simulink model "Flexible_Fishtail_CTLSys"  (R2022b)
settings: Solver=FixedStepAuto  StartTime=0.0  StopTime=12  FixedStep=5e-5  RelTol=1e-3
libraries: slpidlib x3, spsMeanLib x1, rllib x1
settings Model: Creator=acer  LastModifiedBy=10640
settings SolverCC: AlgebraicLoopSolver=TrustRegion
settings DataIOCC: ReturnWorkspaceOutputs=off
settings OptimizationCC: DefaultParameterBehavior=Inlined  UseDivisionForNetSlopeComputation=on  GainParamInheritBuiltInType=on  UseFloatMulNetSlope=on  InlineInvariantSignals=on  EnhancedBackFolding=on  PassReuseOutputArgsAs=Individual arguments  ZeroExternalMemoryAtStartup=off  ZeroInternalMemoryAtStartup=off  EfficientFloat2IntCast=on  OptimizeBlockOrder=speed  DifferentSizesBufferReuse=on  OptimizationCustomize=off  EfficientTunableParamExpr=on
settings DebuggingCC: ParameterTunabilityLossMsg=error  UnconnectedInputMsg=warning  UnconnectedOutputMsg=warning  UnconnectedLineMsg=warning  PregeneratedLibrarySubsystemCodeDiagnostic=none  SFMachineParentedDataDiag=warning  ArithmeticOperatorsInVariantConditions=warning
settings HardwareCC: ProdLongLongMode=on
settings ModelReferenceCC: EnableRefExpFcnMdlSchedulingChecks=on
settings SFSimCC: SimUseLocalCustomCode=off  MATLABDynamicMemAlloc=off  CustomCodeUndefinedFunction=UseInterfaceOnly
settings RTWCC: Description=Embedded Coder  SystemTargetFile=ert.tlc  TemplateMakefile=ert_default_tmf  GenerateReport=on  RTWUseLocalCustomCode=off  LaunchReport=on
settings CodeAppCC: ForceParamTrailComments=on  IgnoreCustomStorageClasses=off  OperatorAnnotations=on  SimulinkDataObjDesc=on  SFDataObjDesc=on  InsertBlockDesc=on
settings ERTTargetCC: TargetLangStandard=C99 (ISO)  GenerateSampleERTMain=on  InlinedParameterPlacement=NonHierarchical  ERTCustomFileTemplate=example_file_process.tlc

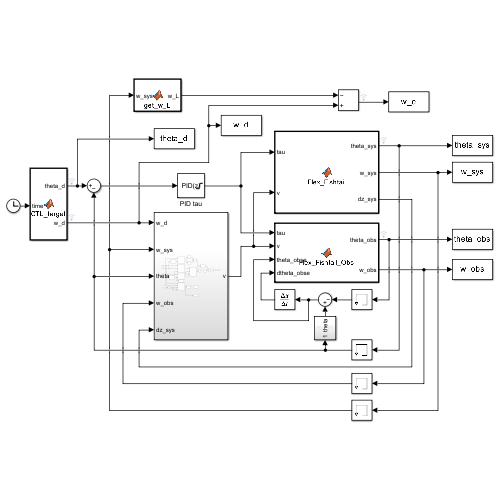
[thumbnail: Simulink's stored preview of the top-level diagram]
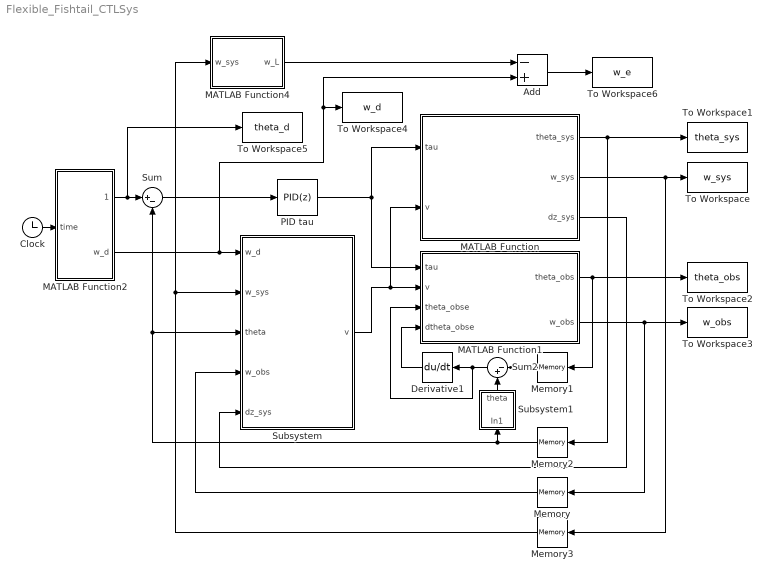
== system Flexible_Fishtail_CTLSys ==
  Add : Sum  Inputs=-+
  Clock : Clock
  Derivative1 : Derivative
  MATLAB Function : MATLAB Function  TreatAsAtomicUnit=on
  MATLAB Function1 : MATLAB Function  TreatAsAtomicUnit=on
  MATLAB Function2 : MATLAB Function  TreatAsAtomicUnit=on
  MATLAB Function4 : MATLAB Function  TreatAsAtomicUnit=on
  Memory{,1..3} (4 alike) : Memory
  PID tau : slpidlib/PID Controller  Controller=PID  Form=Parallel  TimeDomain=Discrete-time  UseExternalTs=off  SampleTime=-1  IntegratorMethod=Forward Euler  FilterMethod=Forward Euler  ControllerParametersSource=internal  P=1.5  I=50  UseKiTs=off  D=0.01  N=100  UseFilter=off  TunerSelectOption=Transfer Function Based (PID Tuner App)  InitialConditionSource=internal  InitialConditionForIntegrator=0  InitialConditionForFilter=0  DifferentiatorICPrevScaledInput=0  ExternalReset=none  TrackingMode=off  Kt=1  LimitOutput=on  SatLimitsSource=internal  UpperSaturationLimit=0.5  LowerSaturationLimit=-0.5  LinearizeAsGain=on  AntiWindupMode=none  Kb=1  LimitIntegrator=off  UpperIntegratorSaturationLimit=inf  LowerIntegratorSaturationLimit=-inf  POutMin=[]  POutMax=[]  IOutMin=[]  IOutMax=[]  DOutMin=[]  DOutMax=[]  NOutMin=[]  NOutMax=[]  SumOutMin=[]  SumOutMax=[]  SaturationOutMin=[]  SaturationOutMax=[]  PParamMin=[]  PParamMax=[]  IParamMin=[]  IParamMax=[]  DParamMin=[]  DParamMax=[]  NParamMin=[]  NParamMax=[]  KbParamMin=[]  KbParamMax=[]  KtParamMin=[]  KtParamMax=[]  KbOutMin=[]  KbOutMax=[]  KtOutMin=[]  KtOutMax=[]  IntegratorOutMin=[]  IntegratorOutMax=[]  FilterOutMin=[]  FilterOutMax=[]  SumI1OutMin=[]  SumI1OutMax=[]  SumI2OutMin=[]  SumI2OutMax=[]  SumI3OutMin=[]  SumI3OutMax=[]  SumI4OutMin=[]  SumI4OutMax=[]  SumDOutMin=[]  SumDOutMax=[]  DifferentiatorOutMin=[]  DifferentiatorOutMax=[]  FilterDiffOutCoefMin=[]  FilterDiffOutCoefMax=[]  ReciprocalOutMin=[]  ReciprocalOutMax=[]  SumDenOutMin=[]  SumDenOutMax=[]  SumNumOutMin=[]  SumNumOutMax=[]  DivideOutMin=[]  DivideOutMax=[]  UdiffTsProdOutMin=[]  UdiffTsProdOutMax=[]  NTsProdOutMin=[]  NTsProdOutMax=[]  UintegralTsProdOutMin=[]  UintegralTsProdOutMax=[]  UngainTsProdOutMin=[]  UngainTsProdOutMax=[]  ClampingZeroOutDataTypeStr=Inherit: Inherit via back propagation  ClampingZeroOutMin=[]  ClampingZeroOutMax=[]  FilterDenConstantOutDataTypeStr=Inherit: Inherit via back propagation  FilterDenConstantOutMin=[]  FilterDenConstantOutMax=[]  PCopyOutDataTypeStr=Inherit: Inherit via back propagation  PCopyOutMin=[]  PCopyOutMax=[]  NCopyOutDataTypeStr=Inherit: Inherit via back propagation  NCopyOutMin=[]  NCopyOutMax=[]  IntegratorContinuousStateAttributes=''  IntegratorStateMustResolveToSignalObject=off  IntegratorRTWStateStorageClass=Auto  FilterContinuousStateAttributes=''  FilterStateMustResolveToSignalObject=off  FilterRTWStateStorageClass=Auto  ParallelPVariant=InternalParameters  IdealPVariant=Disabled  IVariant=InternalParameters  DVariant=InternalParameters  IntegratorVariant=Discrete  SatVariant=Enabled  AWVariant=Passthrough  PCopyVariant=Disabled  TRVariant=Disabled  FdbkBlocksVariant=Forward  IdealPFdbkVariant=Disabled  SatFdbkVariant=Disabled  DerivativeFilterVariant=Differentiator  NVariant=Passthrough  NCopyVariant=Disabled_SignalSpec  FilterICVariant=InternalICsDifferentiator  IntegratorICVariant=InternalICs  ExternalResetVariant=Disabled  TRSumVariant=Passthrough  SumFdbkVariant=Disabled  SumVariant=Sum_PID  TsampFilterVariant=InternalTs  TsampNgainVariant=Passthrough  TsampIntegralVariant=Passthrough  ExternalSaturationOutDataTypeStr=Inherit: Same as second input
  Subsystem : Subsystem
  Subsystem1 : Subsystem
  Sum : Sum  Inputs=|+-
  Sum2 : Sum  Inputs=|-+
  To Workspace : ToWorkspace  VariableName=w_sys  SampleTime=-1
  To Workspace1 : ToWorkspace  VariableName=theta_sys  SampleTime=-1
  To Workspace2 : ToWorkspace  VariableName=theta_obs  SampleTime=-1
  To Workspace3 : ToWorkspace  VariableName=w_obs  SampleTime=-1
  To Workspace4 : ToWorkspace  VariableName=w_d  SampleTime=-1
  To Workspace5 : ToWorkspace  VariableName=theta_d  SampleTime=-1
  To Workspace6 : ToWorkspace  VariableName=w_e  SampleTime=-1
  wires:
  Clock/1 -> MATLAB Function2/1(time)
  MATLAB Function2/1(theta_d) -> To Workspace5/1, Sum/1
  Sum/1 -> PID tau/1
  Derivative1/1 -> MATLAB Function1/4(dtheta_obse)
  MATLAB Function/1(theta_sys) -> Memory2/1, To Workspace1/1
  Sum2/1 -> Derivative1/1, MATLAB Function1/3(theta_obse)
  MATLAB Function2/2(w_d) -> Add/2, To Workspace4/1, Subsystem/1(w_d)
  MATLAB Function1/2(w_obs) -> To Workspace3/1, Memory/1
  MATLAB Function1/1(theta_obs) -> To Workspace2/1, Memory1/1
  Memory1/1 -> Sum2/1
  PID tau/1 -> MATLAB Function/1(tau), MATLAB Function1/1(tau)
  Subsystem/1(v) -> MATLAB Function/2(v), MATLAB Function1/2(v)
  MATLAB Function/2(w_sys) -> Memory3/1, To Workspace/1
  Memory/1 -> Subsystem/4(w_obs)
  Memory2/1 -> Sum/2, Subsystem/3(theta), Subsystem1/1(In1)
  Subsystem1/1(theta) -> Sum2/2
  Memory3/1 -> MATLAB Function4/1(w_sys), Subsystem/2(w_sys)
  MATLAB Function4/1(w_L) -> Add/1
  Add/1 -> To Workspace6/1
  MATLAB Function/3(dz_sys) -> Subsystem/5(dz_sys)

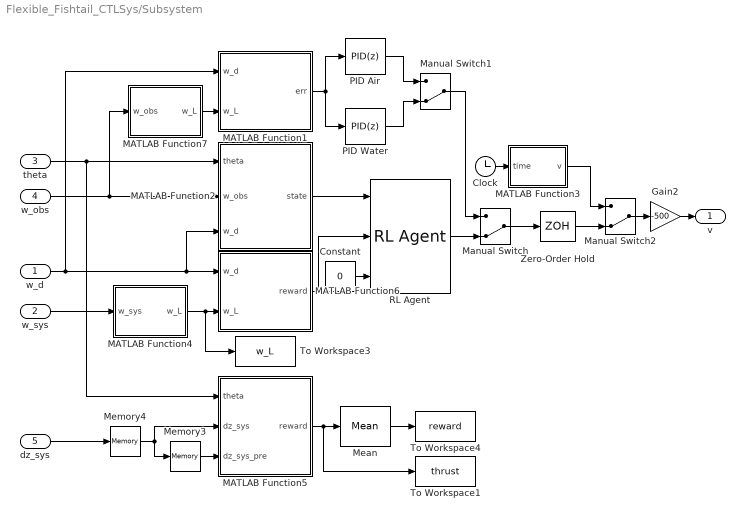
== system Flexible_Fishtail_CTLSys/Subsystem ==
  w_d : Inport
  w_sys : Inport  Port=2
  theta : Inport  Port=3
  w_obs : Inport  Port=4
  dz_sys : Inport  Port=5
  Clock : Clock
  Constant : Constant  Value=0
  Gain2 : Gain  Gain=-500
  MATLAB Function1 : MATLAB Function  TreatAsAtomicUnit=on
  MATLAB Function2 : MATLAB Function  TreatAsAtomicUnit=on
  MATLAB Function3 : MATLAB Function  TreatAsAtomicUnit=on
  MATLAB Function4 : MATLAB Function  TreatAsAtomicUnit=on
  MATLAB Function5 : MATLAB Function  TreatAsAtomicUnit=on
  MATLAB Function6 : MATLAB Function  TreatAsAtomicUnit=on
  MATLAB Function7 : MATLAB Function  TreatAsAtomicUnit=on
  Manual Switch : ManualSwitch  CurrentSetting=0
  Manual Switch1 : ManualSwitch  CurrentSetting=0
  Manual Switch2 : ManualSwitch  CurrentSetting=0
  Mean : spsMeanLib/Mean  Freq=0.5  Vinit=0  Ts=5e-5
  Memory3 : Memory
  Memory4 : Memory
  PID Air : slpidlib/PID Controller  Controller=PID  Form=Parallel  TimeDomain=Discrete-time  UseExternalTs=off  SampleTime=-1  IntegratorMethod=Forward Euler  FilterMethod=Forward Euler  ControllerParametersSource=internal  P=0.00005  I=0.02  UseKiTs=off  D=0  N=100  UseFilter=off  TunerSelectOption=Transfer Function Based (PID Tuner App)  InitialConditionSource=internal  InitialConditionForIntegrator=0  InitialConditionForFilter=0  DifferentiatorICPrevScaledInput=0  ExternalReset=none  TrackingMode=off  Kt=1  LimitOutput=on  SatLimitsSource=internal  UpperSaturationLimit=1  LowerSaturationLimit=-1  LinearizeAsGain=on  AntiWindupMode=none  Kb=1  LimitIntegrator=off  UpperIntegratorSaturationLimit=inf  LowerIntegratorSaturationLimit=-inf  POutMin=[]  POutMax=[]  IOutMin=[]  IOutMax=[]  DOutMin=[]  DOutMax=[]  NOutMin=[]  NOutMax=[]  SumOutMin=[]  SumOutMax=[]  SaturationOutMin=[]  SaturationOutMax=[]  PParamMin=[]  PParamMax=[]  IParamMin=[]  IParamMax=[]  DParamMin=[]  DParamMax=[]  NParamMin=[]  NParamMax=[]  KbParamMin=[]  KbParamMax=[]  KtParamMin=[]  KtParamMax=[]  KbOutMin=[]  KbOutMax=[]  KtOutMin=[]  KtOutMax=[]  IntegratorOutMin=[]  IntegratorOutMax=[]  FilterOutMin=[]  FilterOutMax=[]  SumI1OutMin=[]  SumI1OutMax=[]  SumI2OutMin=[]  SumI2OutMax=[]  SumI3OutMin=[]  SumI3OutMax=[]  SumI4OutMin=[]  SumI4OutMax=[]  SumDOutMin=[]  SumDOutMax=[]  DifferentiatorOutMin=[]  DifferentiatorOutMax=[]  FilterDiffOutCoefMin=[]  FilterDiffOutCoefMax=[]  ReciprocalOutMin=[]  ReciprocalOutMax=[]  SumDenOutMin=[]  SumDenOutMax=[]  SumNumOutMin=[]  SumNumOutMax=[]  DivideOutMin=[]  DivideOutMax=[]  UdiffTsProdOutMin=[]  UdiffTsProdOutMax=[]  NTsProdOutMin=[]  NTsProdOutMax=[]  UintegralTsProdOutMin=[]  UintegralTsProdOutMax=[]  UngainTsProdOutMin=[]  UngainTsProdOutMax=[]  ClampingZeroOutDataTypeStr=Inherit: Inherit via back propagation  ClampingZeroOutMin=[]  ClampingZeroOutMax=[]  FilterDenConstantOutDataTypeStr=Inherit: Inherit via back propagation  FilterDenConstantOutMin=[]  FilterDenConstantOutMax=[]  PCopyOutDataTypeStr=Inherit: Inherit via back propagation  PCopyOutMin=[]  PCopyOutMax=[]  NCopyOutDataTypeStr=Inherit: Inherit via back propagation  NCopyOutMin=[]  NCopyOutMax=[]  IntegratorContinuousStateAttributes=''  IntegratorStateMustResolveToSignalObject=off  IntegratorRTWStateStorageClass=Auto  FilterContinuousStateAttributes=''  FilterStateMustResolveToSignalObject=off  FilterRTWStateStorageClass=Auto  ParallelPVariant=InternalParameters  IdealPVariant=Disabled  IVariant=InternalParameters  DVariant=InternalParameters  IntegratorVariant=Discrete  SatVariant=Enabled  AWVariant=Passthrough  PCopyVariant=Disabled  TRVariant=Disabled  FdbkBlocksVariant=Forward  IdealPFdbkVariant=Disabled  SatFdbkVariant=Disabled  DerivativeFilterVariant=Differentiator  NVariant=Passthrough  NCopyVariant=Disabled_SignalSpec  FilterICVariant=InternalICsDifferentiator  IntegratorICVariant=InternalICs  ExternalResetVariant=Disabled  TRSumVariant=Passthrough  SumFdbkVariant=Disabled  SumVariant=Sum_PID  TsampFilterVariant=InternalTs  TsampNgainVariant=Passthrough  TsampIntegralVariant=Passthrough  ExternalSaturationOutDataTypeStr=Inherit: Same as second input
  PID Water : slpidlib/PID Controller  Controller=PID  Form=Parallel  TimeDomain=Discrete-time  UseExternalTs=off  SampleTime=-1  IntegratorMethod=Forward Euler  FilterMethod=Forward Euler  ControllerParametersSource=internal  P=0.0001  I=0.035  UseKiTs=off  D=0.00000001  N=100  UseFilter=off  TunerSelectOption=Transfer Function Based (PID Tuner App)  InitialConditionSource=internal  InitialConditionForIntegrator=0  InitialConditionForFilter=0  DifferentiatorICPrevScaledInput=0  ExternalReset=none  TrackingMode=off  Kt=1  LimitOutput=on  SatLimitsSource=internal  UpperSaturationLimit=1  LowerSaturationLimit=-1  LinearizeAsGain=on  AntiWindupMode=none  Kb=1  LimitIntegrator=off  UpperIntegratorSaturationLimit=inf  LowerIntegratorSaturationLimit=-inf  POutMin=[]  POutMax=[]  IOutMin=[]  IOutMax=[]  DOutMin=[]  DOutMax=[]  NOutMin=[]  NOutMax=[]  SumOutMin=[]  SumOutMax=[]  SaturationOutMin=[]  SaturationOutMax=[]  PParamMin=[]  PParamMax=[]  IParamMin=[]  IParamMax=[]  DParamMin=[]  DParamMax=[]  NParamMin=[]  NParamMax=[]  KbParamMin=[]  KbParamMax=[]  KtParamMin=[]  KtParamMax=[]  KbOutMin=[]  KbOutMax=[]  KtOutMin=[]  KtOutMax=[]  IntegratorOutMin=[]  IntegratorOutMax=[]  FilterOutMin=[]  FilterOutMax=[]  SumI1OutMin=[]  SumI1OutMax=[]  SumI2OutMin=[]  SumI2OutMax=[]  SumI3OutMin=[]  SumI3OutMax=[]  SumI4OutMin=[]  SumI4OutMax=[]  SumDOutMin=[]  SumDOutMax=[]  DifferentiatorOutMin=[]  DifferentiatorOutMax=[]  FilterDiffOutCoefMin=[]  FilterDiffOutCoefMax=[]  ReciprocalOutMin=[]  ReciprocalOutMax=[]  SumDenOutMin=[]  SumDenOutMax=[]  SumNumOutMin=[]  SumNumOutMax=[]  DivideOutMin=[]  DivideOutMax=[]  UdiffTsProdOutMin=[]  UdiffTsProdOutMax=[]  NTsProdOutMin=[]  NTsProdOutMax=[]  UintegralTsProdOutMin=[]  UintegralTsProdOutMax=[]  UngainTsProdOutMin=[]  UngainTsProdOutMax=[]  ClampingZeroOutDataTypeStr=Inherit: Inherit via back propagation  ClampingZeroOutMin=[]  ClampingZeroOutMax=[]  FilterDenConstantOutDataTypeStr=Inherit: Inherit via back propagation  FilterDenConstantOutMin=[]  FilterDenConstantOutMax=[]  PCopyOutDataTypeStr=Inherit: Inherit via back propagation  PCopyOutMin=[]  PCopyOutMax=[]  NCopyOutDataTypeStr=Inherit: Inherit via back propagation  NCopyOutMin=[]  NCopyOutMax=[]  IntegratorContinuousStateAttributes=''  IntegratorStateMustResolveToSignalObject=off  IntegratorRTWStateStorageClass=Auto  FilterContinuousStateAttributes=''  FilterStateMustResolveToSignalObject=off  FilterRTWStateStorageClass=Auto  ParallelPVariant=InternalParameters  IdealPVariant=Disabled  IVariant=InternalParameters  DVariant=InternalParameters  IntegratorVariant=Discrete  SatVariant=Enabled  AWVariant=Passthrough  PCopyVariant=Disabled  TRVariant=Disabled  FdbkBlocksVariant=Forward  IdealPFdbkVariant=Disabled  SatFdbkVariant=Disabled  DerivativeFilterVariant=Differentiator  NVariant=Passthrough  NCopyVariant=Disabled_SignalSpec  FilterICVariant=InternalICsDifferentiator  IntegratorICVariant=InternalICs  ExternalResetVariant=Disabled  TRSumVariant=Passthrough  SumFdbkVariant=Disabled  SumVariant=Sum_PID  TsampFilterVariant=InternalTs  TsampNgainVariant=Passthrough  TsampIntegralVariant=Passthrough  ExternalSaturationOutDataTypeStr=Inherit: Same as second input
  RL Agent : rllib/RL Agent  Agent=agent  ExternalActionAsInput=off  ProvideLastAction=off  ProvideCumRwd=off  TreatAsDirectFeedthrough=on  UseStrictObservationDataTypes=off
  To Workspace1 : ToWorkspace  VariableName=thrust  SampleTime=-1
  To Workspace3 : ToWorkspace  VariableName=w_L  SampleTime=-1
  To Workspace4 : ToWorkspace  VariableName=reward  SampleTime=-1
  Zero-Order Hold : ZeroOrderHold  SampleTime=20e-3
  v : Outport  VectorParamsAs1DForOutWhenUnconnected=off
  wires:
  Memory3/1 -> MATLAB Function5/3(dz_sys_pre)
  Memory4/1 -> Memory3/1, MATLAB Function5/2(dz_sys)
  Constant/1 -> RL Agent/3
  w_d/1 -> MATLAB Function1/1(w_d), MATLAB Function2/3(w_d), MATLAB Function6/1(w_d)
  w_sys/1 -> MATLAB Function4/1(w_sys)
  w_obs/1 -> MATLAB Function7/1(w_obs), MATLAB Function2/2(w_obs)
  RL Agent/1 -> Manual Switch/2
  MATLAB Function1/1(err) -> PID Water/1, PID Air/1
  MATLAB Function2/1(state) -> RL Agent/1
  MATLAB Function6/1(reward) -> RL Agent/2
  Gain2/1 -> v/1
  Mean/1 -> To Workspace4/1
  PID Air/1 -> Manual Switch1/1
  Manual Switch1/1 -> Manual Switch/1
  PID Water/1 -> Manual Switch1/2
  Clock/1 -> MATLAB Function3/1(time)
  MATLAB Function4/1(w_L) -> To Workspace3/1, MATLAB Function6/2(w_L)
  MATLAB Function7/1(w_L) -> MATLAB Function1/2(w_L)
  Manual Switch/1 -> Zero-Order Hold/1
  Zero-Order Hold/1 -> Manual Switch2/2
  MATLAB Function3/1(v) -> Manual Switch2/1
  Manual Switch2/1 -> Gain2/1
  MATLAB Function5/1(reward) -> To Workspace1/1, Mean/1
  dz_sys/1 -> Memory4/1
  theta/1 -> MATLAB Function5/1(theta), MATLAB Function2/1(theta)

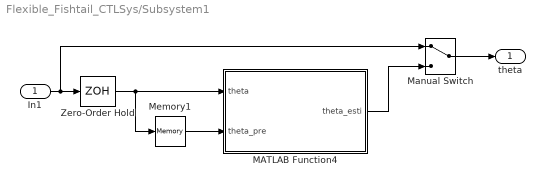
== system Flexible_Fishtail_CTLSys/Subsystem1 ==
  In1 : Inport
  MATLAB Function4 : MATLAB Function  TreatAsAtomicUnit=on
  Manual Switch : ManualSwitch
  Memory1 : Memory
  Zero-Order Hold : ZeroOrderHold  SampleTime=30e-3
  theta : Outport
  wires:
  In1/1 -> Manual Switch/1, Zero-Order Hold/1
  Zero-Order Hold/1 -> MATLAB Function4/1(theta), Memory1/1
  Memory1/1 -> MATLAB Function4/2(theta_pre)
  MATLAB Function4/1(theta_esti) -> Manual Switch/2
  Manual Switch/1 -> theta/1

== matlab function Flexible_Fishtail_CTLSys/Subsystem/MATLAB Function7 ==
  data: w_obs input; w_L output
function w_L = get_w_L(w_obs)
    w_L = w_obs(end);
end

== matlab function Flexible_Fishtail_CTLSys/Subsystem/MATLAB Function4 ==
  data: w_sys input; w_L output
function w_L = get_w_L(w_sys)
    w_L = w_sys(end);
end

== matlab function Flexible_Fishtail_CTLSys/MATLAB Function4 ==
  data: w_sys input; w_L output
function w_L = get_w_L(w_sys)
    w_L = w_sys(end);
end

== matlab function Flexible_Fishtail_CTLSys/MATLAB Function1 ==
  settings: updateMethod=DISCRETE
  data: theta_obs output; w_obs output; tau input; v input; theta_obse input; dtheta_obse input
function [theta_obs, w_obs] = Flex_Fishtail_Obs(tau, v, theta_obse, dtheta_obse)
    %***********************************************************
    persistent angle_obs;
    persistent angle_obs_pre;
    persistent omega_obs;
    persistent omega_obs_pre;
    
    if isempty(angle_obs)
        angle_obs = 10/180*pi;
        angle_obs_pre = angle_obs;
        omega_obs = [ 0; 0; 0; 0; 0; 0; 0; 0; 0; 0; 0; 0; 0; 0; 0; 0; 0; 0; 0];
        omega_obs_pre = omega_obs;
    end
    
    dt = 5e-5;
    
    k_obs=0.015;
    gamma_obs=15;

    Ih=1e-6;
    c=0.1;
    rhow=1000;
    Caf=0.05;
    Cdf=1.2;

    L=0.17;
    nx=19;
    dx=L/(nx-1);
    bx1=round(0.03/dx)+1;
    bx2=round(0.14/dx)+1;
    xL0=round(0.0365/dx)+1;
    xL1=round(0.1375/dx)+1;

    d=0.0002;
    Eb=230e9;
    rhob=1760;
    dmfc=0.0003;
    bmfc=0.014;
    Emfc=30.336e9;
    rhoc=5440;
    d33=460e-12;
    deltad=0.5e-3;
    b=zeros(nx,1);
    EI=zeros(nx,1);
    rho_w=zeros(nx,1);
    cw=zeros(nx,1);
    rho=zeros(nx,1);
    R=zeros(nx,1);

    elecmech=1.66*2*Emfc*bmfc*d33*(d*dmfc+dmfc^2)/(2*deltad);

    for i=1:nx
        if i<bx1
            b(i)=0.04;
        elseif i>bx2
            b(i)=2.3*(i-bx2)*dx+0.026;
        else
            b(i)=2*sqrt(0.96375^2-((i-bx1)*dx)^2)-1.8875;
        end
    end

    for i=1:nx
        if i<xL0
            R(i)=0;
        elseif i>xL1
            R(i)=0;
        else
            R(i)=1;
        end
        EI(i)=R(i)*Emfc*bmfc*(2*dmfc^3/3+d*dmfc^2+0.5*dmfc*d^2)+Eb*d^3*b(i)/12;
        rho_w(i)=0.25*pi*rhow*b(i)^2*Caf;
        cw(i)=0.5*rhow*b(i)*Cdf;
        rho(i)=R(i)*dmfc*bmfc*2*rhoc+d*b(i)*rhob+rho_w(i);
    end
    
    theta=angle_obs;
    theta_pre=angle_obs_pre;
    w=omega_obs;
    w_pre=omega_obs_pre;

    w_new=zeros(nx,1);
    dw=zeros(nx,1);
    dz=zeros(nx,1);
    wxx=zeros(nx,1);
    EIwxx=zeros(nx,1);
    MR=zeros(nx,1);
        
    wxx0=(w(bx1+1)-2*w(bx1)+w(bx1-1))/dx^2;
    theta_new=2*theta-theta_pre+(EI(1)*wxx0+tau...
              +k_obs*(dtheta_obse+gamma_obs*theta_obse)...
              +gamma_obs*Ih*dtheta_obse)*dt^2/Ih;
    
    dtheta=(theta-theta_pre)/dt;
    ddtheta=(theta_new-2*theta+theta_pre)/dt^2;
    for i=1:nx
        dw(i)=(w(i)-w_pre(i))/dt;
        dz(i)=(i-1)*dx*dtheta+dw(i);
    end
    for i=2:nx-1
        wxx(i)=(w(i+1)-2*w(i)+w(i-1))/dx^2;
        EIwxx(i)=EI(i)*wxx(i);
        MR(i)=elecmech*v*R(i);
    end
    
    %Firstly, 1≤i≤bx1
    for i=1:bx1
        w_new(i)=0;
    end
    
    %Secondly, bx1≤i≤nx-2
    for i=bx1+1:nx-2
        EIwxxxx=(EIwxx(i+1)-2*EIwxx(i)+EIwxx(i-1))/dx^2;
        MRxx=(MR(i+1)-2*MR(i)+MR(i-1))/dx^2;
        w_new(i)=2*w(i)-w_pre(i)+(MRxx-EIwxxxx-c*dz(i)...
...%                  -cw(i)*abs(dz(i))*dz(i)...
                 -rho(i)*(i-1)*dx*ddtheta)*dt^2/rho(i);
    end
    %Thirdly, i=nx-1
    EIwxxxx1=EI(nx-1)*(-2*w(nx)+5*w(nx-1)-4*w(nx-2)+w(nx-3))/dx^4;
    w_new(nx-1)=2*w(nx-1)-w_pre(nx-1)+(-EIwxxxx1-c*dz(nx-1)...
...%                 -cw(nx-1)*abs(dz(nx-1))*dz(nx-1)...
                -rho(nx-1)*(nx-2)*dx*ddtheta)*dt^2/rho(nx-1);
    %Finally, i=nx
    EIwxxxx2=EI(nx)*(2*w(nx)-3*w(nx-1)+w(nx-2))/dx^4;
    w_new(nx)=2*w(nx)-w_pre(nx)+(-EIwxxxx2-c*dz(nx)...
...%                 -cw(nx)*abs(dz(nx))*dz(nx)...
                -rho(nx)*(nx-1)*dx*ddtheta)*dt^2/rho(nx);
       
    angle_obs=theta_new;
    angle_obs_pre=theta;
    omega_obs=w_new;
    omega_obs_pre=w;
    
    theta_obs=theta_new;
    w_obs=w_new;
    
end

== matlab function Flexible_Fishtail_CTLSys/MATLAB Function ==
  settings: updateMethod=DISCRETE
  data: theta_sys output; w_sys output; tau input; v input; dz_sys output
function [theta_sys, w_sys, dz_sys] = Flex_Fishtail(tau, v)
    %***********************************************************
    persistent angle;
    persistent angle_pre;
    persistent omega;
    persistent omega_pre;
    
    if isempty(angle)
%         angle = (2 * rand() - 1)*5/180*pi;
        angle = 10/180*pi;
        angle_pre = angle;
%         omega = [ 0; 0; -0.0002; -0.0004;
%             -0.0007; -0.0011; -0.0016; -0.0022;
%             -0.0029; -0.0036; -0.0045; -0.0054;
%             -0.0064; -0.0075; -0.0087; -0.0100;
%             -0.0114; -0.0129; -0.0145];
        omega = [ 0; 0; 0; 0; 0; 0; 0; 0; 0; 0; 0; 0; 0; 0; 0; 0; 0; 0; 0];
        omega_pre = omega;
    end
    
    dt = 5e-5;

    Ih=1e-6;
    c=0.1;
    rhow=1000;
    Caf=0.05;
    Cdf=1.2;

    L=0.17;
    nx=19;
    dx=L/(nx-1);
    bx1=round(0.03/dx)+1;
    bx2=round(0.14/dx)+1;
    xL0=round(0.0365/dx)+1;
    xL1=round(0.1375/dx)+1;

    d=0.0002;
    Eb=230e9;
    rhob=1760;
    dmfc=0.0003;
    bmfc=0.014;
    Emfc=30.336e9;
    rhoc=5440;
    d33=460e-12;
    deltad=0.5e-3;
    b=zeros(nx,1);
    EI=zeros(nx,1);
    rho_w=zeros(nx,1);
    cw=zeros(nx,1);
    rho=zeros(nx,1);
    R=zeros(nx,1);

    elecmech=1.66*2*Emfc*bmfc*d33*(d*dmfc+dmfc^2)/(2*deltad);

    for i=1:nx
        if i<bx1
            b(i)=0.04;
        elseif i>bx2
            b(i)=2.3*(i-bx2)*dx+0.026;
        else
            b(i)=2*sqrt(0.96375^2-((i-bx1)*dx)^2)-1.8875;
        end
    end

    for i=1:nx
        if i<xL0
            R(i)=0;
        elseif i>xL1
            R(i)=0;
        else
            R(i)=1;
        end
        EI(i)=R(i)*Emfc*bmfc*(2*dmfc^3/3+d*dmfc^2+0.5*dmfc*d^2)+Eb*d^3*b(i)/12;
        rho_w(i)=0.25*pi*rhow*b(i)^2*Caf;
        cw(i)=0.5*rhow*b(i)*Cdf;
        rho(i)=R(i)*dmfc*bmfc*2*rhoc+d*b(i)*rhob+rho_w(i);
    end
    
    theta=angle;
    theta_pre=angle_pre;
    w=omega;
    w_pre=omega_pre;

    w_new=zeros(nx,1);
    dw=zeros(nx,1);
    dz=zeros(nx,1);
    wxx=zeros(nx,1);
    EIwxx=zeros(nx,1);
    MR=zeros(nx,1);
        
    wxx0=(w(bx1+1)-2*w(bx1)+w(bx1-1))/dx^2;
    theta_new=2*theta-theta_pre+(EI(1)*wxx0+tau)*dt^2/Ih;
    
    dtheta=(theta-theta_pre)/dt;
    ddtheta=(theta_new-2*theta+theta_pre)/dt^2;
    for i=1:nx
        dw(i)=(w(i)-w_pre(i))/dt;
        dz(i)=(i-1)*dx*dtheta+dw(i);
    end
    for i=2:nx-1
        wxx(i)=(w(i+1)-2*w(i)+w(i-1))/dx^2;
        EIwxx(i)=EI(i)*wxx(i);
        MR(i)=elecmech*v*R(i);
    end
    
    %Firstly, 1≤i≤bx1
    for i=1:bx1
        w_new(i)=0;
    end
    
    %Secondly, bx1≤i≤nx-2
    for i=bx1+1:nx-2
        EIwxxxx=(EIwxx(i+1)-2*EIwxx(i)+EIwxx(i-1))/dx^2;
        MRxx=(MR(i+1)-2*MR(i)+MR(i-1))/dx^2;
        w_new(i)=2*w(i)-w_pre(i)+(MRxx-EIwxxxx-c*dz(i)...
                 -cw(i)*abs(dz(i))*dz(i)...
                 -rho(i)*(i-1)*dx*ddtheta)*dt^2/rho(i);
    end
    %Thirdly, i=nx-1
    EIwxxxx1=EI(nx-1)*(-2*w(nx)+5*w(nx-1)-4*w(nx-2)+w(nx-3))/dx^4;
    w_new(nx-1)=2*w(nx-1)-w_pre(nx-1)+(-EIwxxxx1-c*dz(nx-1)...
                -cw(nx-1)*abs(dz(nx-1))*dz(nx-1)...
                -rho(nx-1)*(nx-2)*dx*ddtheta)*dt^2/rho(nx-1);
    %Finally, i=nx
    EIwxxxx2=EI(nx)*(2*w(nx)-3*w(nx-1)+w(nx-2))/dx^4;
    w_new(nx)=2*w(nx)-w_pre(nx)+(-EIwxxxx2-c*dz(nx)...
                -cw(nx)*abs(dz(nx))*dz(nx)...
                -rho(nx)*(nx-1)*dx*ddtheta)*dt^2/rho(nx);
       
    angle=theta_new;
    angle_pre=theta;
    omega=w_new;
    omega_pre=w;
    
    theta_sys=theta_new;
    w_sys=w_new;
    dz_sys=dz;
end

== matlab function Flexible_Fishtail_CTLSys/MATLAB Function2 ==
  settings: updateMethod=DISCRETE
  data: theta_d output; w_d output; time input
function [theta_d, w_d] = CTL_target(time)
    c1=10/180*pi;
    c2=0.01;
    L=0.17;
    lamda=L*50;

    amp = 0.004;
    phase = 0;

    if time < 8
        f = 0.5;
    else
        f = 1.0;
    end
    
    theta_d=c1*sin(2*pi*f*time);
%     theta_d=c1;
%     theta_d = 0;
    w_d=(c1*L+c2*L^2)*sin(2*pi*(f*time+L/lamda))-L*theta_d;
%     w_d=amp*sin(2*pi*(f*time+phase/360));
%     w_d=0;

end

== matlab function Flexible_Fishtail_CTLSys/Subsystem/MATLAB Function3 ==
  settings: updateMethod=DISCRETE
  data: v output; time input
function v  = CTL_target(time)

%     if time<10
%         f = 0.5;
%     elseif time>=10 && time<15
%         f = 1.0;
%     else
%         f = 1.5;
%     end

    f = 1;
    
    v=sin(2*pi*f*time);

end

== matlab function Flexible_Fishtail_CTLSys/Subsystem/MATLAB Function1 ==
  data: w_d input; err output; w_L input
function err = Get_Error(w_d, w_L)

    err = w_d - w_L;
    ke = 1e5;

    err = ke * err;

end

== matlab function Flexible_Fishtail_CTLSys/Subsystem/MATLAB Function5 ==
  data: theta input; dz_sys input; reward output; dz_sys_pre input
function reward = Get_Reward(theta, dz_sys, dz_sys_pre)
    dt = 5e-5;

    rhow=1000;
    Caf=0.05;
    Cdf=1.2;

    L=0.17;
    nx=19;
    dx=L/(nx-1);
    bx1=round(0.03/dx)+1;
    bx2=round(0.14/dx)+1;

    b=zeros(nx,1);
    rho_w=zeros(nx,1);
    cw=zeros(nx,1);
    
    for i=1:nx
        if i<bx1
            b(i)=0.04;
        elseif i>bx2
            b(i)=2.3*(i-bx2)*dx+0.026;
        else
            b(i)=2*sqrt(0.96375^2-((i-bx1)*dx)^2)-1.8875;
        end
    end

    for i=1:nx
        rho_w(i)=0.25*pi*rhow*b(i)^2*Caf;
        cw(i)=0.5*rhow*b(i)*Cdf;
    end

    reward=-dx*(cw(1)*abs(dz_sys(1))*dz_sys(1)+...
               rho_w(1)*(dz_sys(1)-dz_sys_pre(1))/dt)*theta;
    for i=2:nx
        reward=reward-dx*(cw(i)*abs(dz_sys(i))*dz_sys(i)+...
               rho_w(i)*(dz_sys(i)-dz_sys_pre(i))/dt)*theta;
    end
end

== matlab function Flexible_Fishtail_CTLSys/Subsystem/MATLAB Function6 ==
  data: w_d input; reward output; w_L input
function reward = Get_Reward(w_d, w_L)

    err = w_d - w_L;
    ke = 1e4;

    reward = -ke*err*err;

end

== matlab function Flexible_Fishtail_CTLSys/Subsystem1/MATLAB Function4 ==
  data: theta input; theta_esti output; theta_pre input
function theta_esti = theta_estimation(theta,theta_pre)
    persistent theta_esti_preval;
    persistent theta_esti_val;
    persistent obs_cal_count;
    persistent obs_record;

    if isempty(obs_cal_count)
        theta_esti_preval = 0;
        theta_esti_val = 0;
        obs_cal_count = 0;
        obs_record = 0;
    end

    dt_obs = 5e-5;    
    dt_fb = 30e-3;
    obs_cal_count = obs_cal_count + 1;

    if theta ~= theta_pre
        theta_esti_preval = theta_pre;
        theta_esti_val = theta;
        obs_record = obs_cal_count;
    end

    theta_esti = theta_esti_preval + (theta_esti_val - theta_esti_preval) / dt_fb ...
                                * (obs_cal_count-obs_record) * dt_obs;
%     theta_esti = interp1([0 dt_fb],[theta_esti_preval theta_esti_val],(obs_cal_count - obs_record)*dt_obs,'spline');

end

== matlab function Flexible_Fishtail_CTLSys/Subsystem/MATLAB Function2 ==
  data: theta input; w_obs input; state output; w_d input
function state = Get_State(theta, w_obs, w_d)

    state = [theta;
             w_obs(9);
             w_obs(14);
             w_obs(end);
             w_d];

end
